simulink model "SIL_OlfatiSaber"  (R2021b)
settings: Solver=FixedStepDiscrete  StartTime=0  StopTime=T  FixedStep=0.01  RelTol=1e-3  EnableMultiTasking=on
model workspace (MAT data in the model file):
  SL_ROS_VariableLengthArrays_MaxSizes.CommonInfo.ArrayTruncateAction = 'EmitWarning'
  SL_ROS_VariableLengthArrays_MaxSizes.MsgTypeMap = containers.Map
  SL_ROS_VariableLengthArrays_MaxSizes.MsgTypeMap.serialization.keys = {'aircraft_communication/NetworkComm', 'aircraft_messages/Communication', 'aircraft_messages/NetworkComm', 'cosmus_messages/Communication', 'cosmus_messages/NetworkComm', 'cosmus_messages/WifiSignal', 'cosmus_messages/WifiSignals', 'sensor_msgs/Image'}
  SL_ROS_VariableLengthArrays_MaxSizes.MsgTypeMap.serialization.values{1}.PropertyName = 'Comms'
  SL_ROS_VariableLengthArrays_MaxSizes.MsgTypeMap.serialization.values{1}.DataType = 'aircraft_communication/Communication'
  SL_ROS_VariableLengthArrays_MaxSizes.MsgTypeMap.serialization.values{1}.MaxLength = 4
  SL_ROS_VariableLengthArrays_MaxSizes.MsgTypeMap.serialization.values{2}.PropertyName = 'Ssid'
  SL_ROS_VariableLengthArrays_MaxSizes.MsgTypeMap.serialization.values{2}.DataType = 'uint8'
  SL_ROS_VariableLengthArrays_MaxSizes.MsgTypeMap.serialization.values{2}.MaxLength = 6
  SL_ROS_VariableLengthArrays_MaxSizes.MsgTypeMap.serialization.values{3}.PropertyName = 'Comms'
  SL_ROS_VariableLengthArrays_MaxSizes.MsgTypeMap.serialization.values{3}.DataType = 'aircraft_messages/Communication'
  SL_ROS_VariableLengthArrays_MaxSizes.MsgTypeMap.serialization.values{3}.MaxLength = 4
  SL_ROS_VariableLengthArrays_MaxSizes.MsgTypeMap.serialization.values{4}.PropertyName = 'Ssid'
  SL_ROS_VariableLengthArrays_MaxSizes.MsgTypeMap.serialization.values{4}.DataType = 'uint8'
  SL_ROS_VariableLengthArrays_MaxSizes.MsgTypeMap.serialization.values{4}.MaxLength = 16
  SL_ROS_VariableLengthArrays_MaxSizes.MsgTypeMap.serialization.values{5}.PropertyName = 'Comms'
  SL_ROS_VariableLengthArrays_MaxSizes.MsgTypeMap.serialization.values{5}.DataType = 'cosmus_messages/Communication'
  SL_ROS_VariableLengthArrays_MaxSizes.MsgTypeMap.serialization.values{5}.MaxLength = 5
  SL_ROS_VariableLengthArrays_MaxSizes.MsgTypeMap.serialization.values{6}.PropertyName = 'Ssid'
  SL_ROS_VariableLengthArrays_MaxSizes.MsgTypeMap.serialization.values{6}.DataType = 'uint8'
  SL_ROS_VariableLengthArrays_MaxSizes.MsgTypeMap.serialization.values{6}.MaxLength = 1
  SL_ROS_VariableLengthArrays_MaxSizes.MsgTypeMap.serialization.values{7}.PropertyName = 'Signals'
  SL_ROS_VariableLengthArrays_MaxSizes.MsgTypeMap.serialization.values{7}.DataType = 'cosmus_messages/WifiSignal'
  SL_ROS_VariableLengthArrays_MaxSizes.MsgTypeMap.serialization.values{7}.MaxLength = 5
  SL_ROS_VariableLengthArrays_MaxSizes.MsgTypeMap.serialization.values{8}(1).PropertyName = 'Data'
  SL_ROS_VariableLengthArrays_MaxSizes.MsgTypeMap.serialization.values{8}(1).DataType = 'uint8'
  SL_ROS_VariableLengthArrays_MaxSizes.MsgTypeMap.serialization.values{8}(1).MaxLength = 259200
  SL_ROS_VariableLengthArrays_MaxSizes.MsgTypeMap.serialization.values{8}(2).PropertyName = 'Encoding'
  SL_ROS_VariableLengthArrays_MaxSizes.MsgTypeMap.serialization.values{8}(2).DataType = 'uint8'
  SL_ROS_VariableLengthArrays_MaxSizes.MsgTypeMap.serialization.values{8}(2).MaxLength = 259200
  SL_ROS_VariableLengthArrays_MaxSizes.MsgTypeMap.serialization.uniformity = 0
  SL_ROS_VariableLengthArrays_MaxSizes.MsgTypeMap.serialization.keyType = 'char'
  SL_ROS_VariableLengthArrays_MaxSizes.MsgTypeMap.serialization.valueType = 'any'
values from neighbouring files (symbols this model uses):
  airspeed_ref = 42    [start_swarm.m]
  altitude_ref = 300    [start_swarm.m]
  N_Waypoints = size(Waypoints,1)    [start_swarm.m]
  radius_waypoint = 200    [start_swarm.m]
  Waypoints = [1200 -1000 ... (first row only)    [start_swarm.m]
undefined symbols (not defined in the file or in its folder): DiscIntNeverNeededParam, Elevators, p_swarm, Propeller, RightAileron, RightFlap, Rudder
libraries: robotlib x36, slpidlib x15, eeGeneralControl x5, simulink x5
(part 1 of 5)
settings Model: Creator=fcsou  LastModifiedBy=fabricio
settings SolverCC: AlgebraicLoopSolver=TrustRegion
settings OptimizationCC: EnhancedBackFolding=on  PassReuseOutputArgsThreshold=0  MaxStackSize=64  OptimizeBlockOrder=speed  DifferentSizesBufferReuse=on  OptimizationCustomize=off
settings DebuggingCC: ParameterTunabilityLossMsg=error  SFMachineParentedDataDiag=warning
settings HardwareCC: ProdBitPerPointer=32  ProdBitPerSizeT=32  ProdBitPerPtrDiffT=32  ProdLargestAtomicFloat=None  ProdIntDivRoundTo=Undefined  ProdEndianess=Unspecified  ProdWordSize=32  ProdHWDeviceType=Generic->Unspecified (assume 32-bit Generic)  UseEmbeddedCoderFeatures=off
settings SFSimCC: MATLABDynamicMemAlloc=off
settings RTWCC: Description=Embedded Coder  SystemTargetFile=ert.tlc  HardwareBoard=Robot Operating System (ROS)  TLCOptions="-aInlineSetEventsForThisBaseRateFcn=TLC_FALSE -aSuppressMultiTaskScheduler=TLC_FALSE  -aRateBasedStepFcn=0"  TemplateMakefile=ert_default_tmf  Toolchain=Catkin  TargetLang=C++
settings CodeAppCC: ForceParamTrailComments=on  OperatorAnnotations=on
settings ERTTargetCC: ERTCustomFileBanners=off  SupportContinuousTime=on  SupportNonInlinedSFcns=on  RemoveResetFunc=off  ModelStepFunctionPrototypeControlCompliant=off  ERTCustomFileTemplate=rostime_codertarget_file_process.tlc

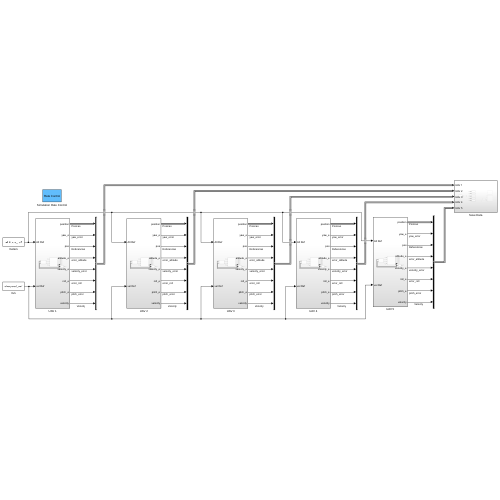
[thumbnail: Simulink's stored preview of the top-level diagram]
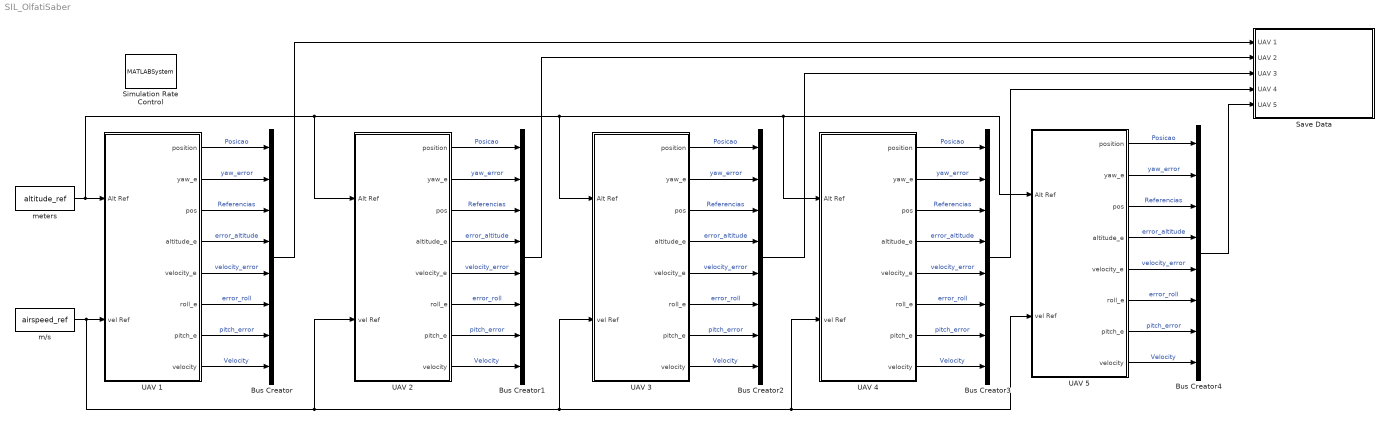
== system SIL_OlfatiSaber ==
  Bus Creator{,1..4} (5 alike) : BusCreator  Inputs=8
  Save Data : Subsystem
  Simulation Rate Control : MATLABSystem  System=ExampleHelperSimulationRateControl  SampleTime=0.01
      mask Type: ExampleHelperSimulationRateControl
      mask Display: disp('Rate Control');
  UAV 1 : Subsystem
  UAV 2 : Subsystem
  UAV 3 : Subsystem
  UAV 4 : Subsystem
  UAV 5 : Subsystem
  m/s : Constant  Value=airspeed_ref
  meters : Constant  Value=altitude_ref
  wires:
  UAV 1/1(position) -> Bus Creator/1  "Posicao"
  UAV 1/2(yaw_e) -> Bus Creator/2  "yaw_error"
  UAV 1/3(pos) -> Bus Creator/3  "Referencias"
  UAV 1/4(altitude_e) -> Bus Creator/4  "error_altitude"
  UAV 1/5(velocity_e) -> Bus Creator/5  "velocity_error"
  UAV 1/6(roll_e) -> Bus Creator/6  "error_roll"
  UAV 1/7(pitch_e) -> Bus Creator/7  "pitch_error"
  m/s/1 -> UAV 5/2(vel Ref), UAV 4/2(vel Ref), UAV 3/2(vel Ref), UAV 2/2(vel Ref), UAV 1/2(vel Ref)
  meters/1 -> UAV 5/1(Alt Ref), UAV 4/1(Alt Ref), UAV 3/1(Alt Ref), UAV 2/1(Alt Ref), UAV 1/1(Alt Ref)
  UAV 1/8(velocity) -> Bus Creator/8  "Velocity"
  UAV 2/7(pitch_e) -> Bus Creator1/7  "pitch_error"
  UAV 2/1(position) -> Bus Creator1/1  "Posicao"
  UAV 2/5(velocity_e) -> Bus Creator1/5  "velocity_error"
  UAV 2/3(pos) -> Bus Creator1/3  "Referencias"
  UAV 2/6(roll_e) -> Bus Creator1/6  "error_roll"
  UAV 2/8(velocity) -> Bus Creator1/8  "Velocity"
  UAV 2/4(altitude_e) -> Bus Creator1/4  "error_altitude"
  UAV 2/2(yaw_e) -> Bus Creator1/2  "yaw_error"
  UAV 3/5(velocity_e) -> Bus Creator2/5  "velocity_error"
  UAV 3/3(pos) -> Bus Creator2/3  "Referencias"
  UAV 3/7(pitch_e) -> Bus Creator2/7  "pitch_error"
  UAV 3/2(yaw_e) -> Bus Creator2/2  "yaw_error"
  UAV 3/6(roll_e) -> Bus Creator2/6  "error_roll"
  UAV 3/4(altitude_e) -> Bus Creator2/4  "error_altitude"
  UAV 3/8(velocity) -> Bus Creator2/8  "Velocity"
  UAV 3/1(position) -> Bus Creator2/1  "Posicao"
  Bus Creator/1 -> Save Data/1(UAV 1)
  Bus Creator1/1 -> Save Data/2(UAV 2)
  Bus Creator2/1 -> Save Data/3(UAV 3)
  UAV 4/4(altitude_e) -> Bus Creator3/4  "error_altitude"
  UAV 4/5(velocity_e) -> Bus Creator3/5  "velocity_error"
  UAV 4/7(pitch_e) -> Bus Creator3/7  "pitch_error"
  UAV 4/8(velocity) -> Bus Creator3/8  "Velocity"
  UAV 4/2(yaw_e) -> Bus Creator3/2  "yaw_error"
  UAV 4/3(pos) -> Bus Creator3/3  "Referencias"
  UAV 4/6(roll_e) -> Bus Creator3/6  "error_roll"
  UAV 4/1(position) -> Bus Creator3/1  "Posicao"
  UAV 5/4(altitude_e) -> Bus Creator4/4  "error_altitude"
  UAV 5/5(velocity_e) -> Bus Creator4/5  "velocity_error"
  UAV 5/7(pitch_e) -> Bus Creator4/7  "pitch_error"
  UAV 5/8(velocity) -> Bus Creator4/8  "Velocity"
  UAV 5/2(yaw_e) -> Bus Creator4/2  "yaw_error"
  UAV 5/3(pos) -> Bus Creator4/3  "Referencias"
  UAV 5/6(roll_e) -> Bus Creator4/6  "error_roll"
  UAV 5/1(position) -> Bus Creator4/1  "Posicao"
  Bus Creator3/1 -> Save Data/4(UAV 4)
  Bus Creator4/1 -> Save Data/5(UAV 5)

== system SIL_OlfatiSaber/Save Data ==
  UAV 1 : Inport
  UAV 2 : Inport  Port=2
  UAV 3 : Inport  Port=3
  UAV 4 : Inport  Port=4
  UAV 5 : Inport  Port=5
  Constant : Constant  Commented=on  Value=p_swarm.r
  Constant1 : Constant  Commented=on  Value=p_swarm.nb_agents
  Current Time : robotlib/Current Time  OutputFormat=double  SampleTime=-1  ModelName=SIL_OlfatiSaber
      settings: SourceProductBaseCode=RR
  Formation Shape Plot : MATLAB Function  Commented=on  TreatAsAtomicUnit=on
  Positions Plot : MATLAB Function  Commented=on  TreatAsAtomicUnit=on
  To Workspace1 : ToWorkspace  VariableName=UAV1  SaveFormat=Timeseries  SampleTime=-1
  To Workspace2 : ToWorkspace  VariableName=UAV2  SaveFormat=Timeseries  SampleTime=-1
  To Workspace3 : ToWorkspace  VariableName=UAV3  SaveFormat=Timeseries  SampleTime=-1
  To Workspace4 : ToWorkspace  VariableName=UAV4  SaveFormat=Timeseries  SampleTime=-1
  To Workspace5 : ToWorkspace  VariableName=UAV5  SaveFormat=Timeseries  SampleTime=-1
  To Workspace6 : ToWorkspace  VariableName=ROStime  SaveFormat=Timeseries  SampleTime=-1
  wires:
  UAV 1/1 -> To Workspace1/1
  UAV 3/1 -> To Workspace3/1
  UAV 4/1 -> To Workspace4/1
  UAV 5/1 -> To Workspace5/1
  Current Time/1 -> To Workspace6/1
  UAV 2/1 -> To Workspace2/1
  Constant/1 -> Formation Shape Plot/3(r_comm)
  Constant1/1 -> Formation Shape Plot/4(max_agent)

== system SIL_OlfatiSaber/UAV 1 ==
  Alt Ref : Inport
  vel Ref : Inport  Port=2
  Filtered Derivative (Discrete or Continuous) : eeGeneralControl/Filtered Derivative (Discrete or Continuous)  K=1  T=0.1  B=inf  A=-inf  minRatio=10  init_option=Inherited from block input  x0=0  Ts=-1
      settings: SourceProductBaseCode=PS
  High-level : Subsystem
  Low-level : Subsystem
  position : Outport
  yaw_e : Outport  Port=2
  pos : Outport  Port=3
  altitude_e : Outport  Port=4
  velocity_e : Outport  Port=5
  roll_e : Outport  Port=6
  pitch_e : Outport  Port=7
  velocity : Outport  Port=8
  wires:
  Low-level/7(position) -> High-level/1(Pos_I), Filtered Derivative (Discrete or Continuous)/1, position/1
  vel Ref/1 -> Low-level/1(vel ref)
  Alt Ref/1 -> Low-level/4(altitude ref)
  Low-level/1(alt_e) -> altitude_e/1
  Low-level/2(yaw_error) -> yaw_e/1
  Low-level/3(positions) -> pos/1
  Low-level/4(vel_e) -> velocity_e/1
  Low-level/5(roll_e) -> roll_e/1
  Low-level/6(pitch_e) -> pitch_e/1
  High-level/1(x ref) -> Low-level/2(x ref)
  High-level/2(y ref) -> Low-level/3(y ref)
  Low-level/8(Network) -> High-level/2(Network_Scan)
  Filtered Derivative (Discrete or Continuous)/1 -> velocity/1

== system SIL_OlfatiSaber/UAV 2 ==
  Alt Ref : Inport
  vel Ref : Inport  Port=2
  Filtered Derivative (Discrete or Continuous) : eeGeneralControl/Filtered Derivative (Discrete or Continuous)  K=1  T=0.1  B=inf  A=-inf  minRatio=10  init_option=Inherited from block input  x0=0  Ts=-1
      settings: SourceProductBaseCode=PS
  High-level : Subsystem
  Low-level : Subsystem
  position : Outport
  yaw_e : Outport  Port=2
  pos : Outport  Port=3
  altitude_e : Outport  Port=4
  velocity_e : Outport  Port=5
  roll_e : Outport  Port=6
  pitch_e : Outport  Port=7
  velocity : Outport  Port=8
  wires:
  Low-level/7(position) -> High-level/1(Pos_I), Filtered Derivative (Discrete or Continuous)/1, position/1
  vel Ref/1 -> Low-level/1(vel ref)
  Alt Ref/1 -> Low-level/4(altitude ref)
  Low-level/1(alt_e) -> altitude_e/1
  Low-level/2(yaw_error) -> yaw_e/1
  Low-level/3(positions) -> pos/1
  Low-level/4(vel_e) -> velocity_e/1
  Low-level/5(roll_e) -> roll_e/1
  Low-level/6(pitch_e) -> pitch_e/1
  High-level/1(x ref) -> Low-level/2(x ref)
  High-level/2(y ref) -> Low-level/3(y ref)
  Low-level/8(Network) -> High-level/2(Network_Scan)
  Filtered Derivative (Discrete or Continuous)/1 -> velocity/1

== system SIL_OlfatiSaber/UAV 3 ==
  Alt Ref : Inport
  vel Ref : Inport  Port=2
  Filtered Derivative (Discrete or Continuous) : eeGeneralControl/Filtered Derivative (Discrete or Continuous)  K=1  T=0.1  B=inf  A=-inf  minRatio=10  init_option=Inherited from block input  x0=0  Ts=-1
      settings: SourceProductBaseCode=PS
  High-level : Subsystem
  Low-level : Subsystem
  position : Outport
  yaw_e : Outport  Port=2
  pos : Outport  Port=3
  altitude_e : Outport  Port=4
  velocity_e : Outport  Port=5
  roll_e : Outport  Port=6
  pitch_e : Outport  Port=7
  velocity : Outport  Port=8
  wires:
  Low-level/7(position) -> Filtered Derivative (Discrete or Continuous)/1, High-level/1(Pos_I), position/1
  vel Ref/1 -> Low-level/1(vel ref)
  Alt Ref/1 -> Low-level/4(altitude ref)
  Low-level/1(alt_e) -> altitude_e/1
  Low-level/2(yaw_error) -> yaw_e/1
  Low-level/3(positions) -> pos/1
  Low-level/4(vel_e) -> velocity_e/1
  Low-level/5(roll_e) -> roll_e/1
  Low-level/6(pitch_e) -> pitch_e/1
  High-level/1(x ref) -> Low-level/2(x ref)
  High-level/2(y ref) -> Low-level/3(y ref)
  Low-level/8(Network) -> High-level/2(Network_Scan)
  Filtered Derivative (Discrete or Continuous)/1 -> velocity/1

== system SIL_OlfatiSaber/UAV 4 ==
  Alt Ref : Inport
  vel Ref : Inport  Port=2
  Filtered Derivative (Discrete or Continuous) : eeGeneralControl/Filtered Derivative (Discrete or Continuous)  K=1  T=0.1  B=inf  A=-inf  minRatio=10  init_option=Inherited from block input  x0=0  Ts=-1
      settings: SourceProductBaseCode=PS
  High-level : Subsystem
  Low-level : Subsystem
  position : Outport
  yaw_e : Outport  Port=2
  pos : Outport  Port=3
  altitude_e : Outport  Port=4
  velocity_e : Outport  Port=5
  roll_e : Outport  Port=6
  pitch_e : Outport  Port=7
  velocity : Outport  Port=8
  wires:
  Low-level/7(position) -> Filtered Derivative (Discrete or Continuous)/1, High-level/1(Pos_I), position/1
  vel Ref/1 -> Low-level/1(vel ref)
  Alt Ref/1 -> Low-level/4(altitude ref)
  Low-level/1(alt_e) -> altitude_e/1
  Low-level/2(yaw_error) -> yaw_e/1
  Low-level/3(positions) -> pos/1
  Low-level/4(vel_e) -> velocity_e/1
  Low-level/5(roll_e) -> roll_e/1
  Low-level/6(pitch_e) -> pitch_e/1
  High-level/1(x ref) -> Low-level/2(x ref)
  High-level/2(y ref) -> Low-level/3(y ref)
  Low-level/8(Network) -> High-level/2(Network_Scan)
  Filtered Derivative (Discrete or Continuous)/1 -> velocity/1

== system SIL_OlfatiSaber/UAV 5 ==
  Alt Ref : Inport
  vel Ref : Inport  Port=2
  Filtered Derivative (Discrete or Continuous) : eeGeneralControl/Filtered Derivative (Discrete or Continuous)  K=1  T=0.1  B=inf  A=-inf  minRatio=10  init_option=Inherited from block input  x0=0  Ts=-1
      settings: SourceProductBaseCode=PS
  High-level : Subsystem
  Low-level : Subsystem
  position : Outport
  yaw_e : Outport  Port=2
  pos : Outport  Port=3
  altitude_e : Outport  Port=4
  velocity_e : Outport  Port=5
  roll_e : Outport  Port=6
  pitch_e : Outport  Port=7
  velocity : Outport  Port=8
  wires:
  Low-level/7(position) -> Filtered Derivative (Discrete or Continuous)/1, High-level/1(Pos_I), position/1
  vel Ref/1 -> Low-level/1(vel ref)
  Alt Ref/1 -> Low-level/4(altitude ref)
  Low-level/1(alt_e) -> altitude_e/1
  Low-level/2(yaw_error) -> yaw_e/1
  Low-level/3(positions) -> pos/1
  Low-level/4(vel_e) -> velocity_e/1
  Low-level/5(roll_e) -> roll_e/1
  Low-level/6(pitch_e) -> pitch_e/1
  High-level/1(x ref) -> Low-level/2(x ref)
  High-level/2(y ref) -> Low-level/3(y ref)
  Low-level/8(Network) -> High-level/2(Network_Scan)
  Filtered Derivative (Discrete or Continuous)/1 -> velocity/1

== system SIL_OlfatiSaber/UAV 1/High-level ==
  Pos_I : Inport
  Network_Scan : Inport  Port=2
  Coordination Algorithm : Subsystem
  Network : Subsystem
  Terminator5 : Terminator
  Waypoint Generator : Subsystem
  x ref : Outport
  y ref : Outport  Port=2
  wires:
  Network/1(Pos_J) -> Coordination Algorithm/1(Xi), Waypoint Generator/1(Xi)
  Network_Scan/1 -> Network/1(Scan)
  Pos_I/1 -> Waypoint Generator/2(Pos_i)
  Coordination Algorithm/1(X) -> x ref/1
  Coordination Algorithm/2(Y) -> y ref/1
  Waypoint Generator/1(u) -> Coordination Algorithm/2(u)
  Coordination Algorithm/3(Z) -> Terminator5/1

== system SIL_OlfatiSaber/UAV 1/Low-level ==
  vel ref : Inport
  x ref : Inport  Port=2
  y ref : Inport  Port=3
  altitude ref : Inport  Port=4
  Autopilot : Subsystem
      settings: PortSchema="{\"entries\":[{\"content\":{\"sides\":[{\"content\":{\"connectorIds\":[\"In1\",\"In2\",\"In3\",\"In4\",\"In5\",\"In6\"]},\"type\":\"ConnectorPlacement.EquallySpacedRectSide\",\"uuid\":\"f5987fb5-26bd-460f-ada3-c62a2cc917d9\"},{\"content\":{\"connectorIds\":[\"Out1\",\"Out2\",\"Out3\",\"Out4\"],\"side\":\"RIGHT\"},\"type\":\"ConnectorPlacement.EquallySpacedRectSide\",\"uuid\":\"78b4fbb6-b2d6-45e8-a79e-ccfb1aa742fa\"},{\"content\":{\"connectorIds\":[\"Out5\",\"Out6\",\"Out7\",\"Out8\"],\"side\":\"TOP\"},\"type\":\"ConnectorPlacement.EquallySpacedRectSide\",\"uuid\":\"043ac8db-db42-42ba-ba46-d4f45f772f93\"},{\"content\":{\"connectorIds\":[],\"side\":\"HIDDEN\"},\"type\":\"ConnectorPlacement.EquallySpacedRectSide\",\"uuid\":\"557a5d68-6739-4613-818d-4b3751c4f08a\"}]},\"type\":\"ConnectorPlacement.EquallySpacedConnector\",\"uuid\":\"675ce67f-dd1b-4b16-8fb4-2c0be5e81414\"}],\"packageUris\":[\"http://schema.mathworks.com/mf0/Connector/R2020b\"],\"version\":\"1.0\"}"
  Bus Selector1 : BusSelector  OutputSignals=PositionX,PositionY
  Guidance Algorithm : Subsystem
      settings: PortSchema="{\"entries\":[{\"content\":{\"sides\":[{\"content\":{\"connectorIds\":[\"In1\",\"In2\",\"In3\",\"In4\",\"In5\"]},\"type\":\"ConnectorPlacement.EquallySpacedRectSide\",\"uuid\":\"b0b83658-dc10-4011-a234-ab17b261f867\"},{\"content\":{\"connectorIds\":[\"Out1\"],\"side\":\"RIGHT\"},\"type\":\"ConnectorPlacement.EquallySpacedRectSide\",\"uuid\":\"f99dae16-3a0a-4b7a-a248-8f98f89ef8fb\"},{\"content\":{\"connectorIds\":[\"Out2\",\"Out3\"],\"side\":\"TOP\"},\"type\":\"ConnectorPlacement.EquallySpacedRectSide\",\"uuid\":\"275bc05e-c915-4930-a6d1-ba5a3a506250\"},{\"content\":{\"connectorIds\":[],\"side\":\"HIDDEN\"},\"type\":\"ConnectorPlacement.EquallySpacedRectSide\",\"uuid\":\"a071ce22-c6e1-49a1-b318-d26a8e8cfe9f\"}]},\"type\":\"ConnectorPlacement.EquallySpacedConnector\",\"uuid\":\"e0998603-dd40-4b43-8488-1ee2e7350a27\"}],\"packageUris\":[\"http://schema.mathworks.com/mf0/Connector/R2020b\"],\"version\":\"1.0\"}"
  ROS Settings : Subsystem
  Vision : Subsystem
  alt_e : Outport
  yaw_error : Outport  Port=2
  positions : Outport  Port=3
  vel_e : Outport  Port=4
  roll_e : Outport  Port=5
  pitch_e : Outport  Port=6
  position : Outport  Port=7
  Network : Outport  Port=8
  wires:
  ROS Settings/2(Yaw) -> Guidance Algorithm/1(yaw)
  ROS Settings/5(velocity) -> Autopilot/5(vel_in)
  Guidance Algorithm/1(roll_ref) -> Autopilot/3(roll_ref)
  ROS Settings/1(Euler angles) -> Autopilot/2(Euler angles)
  Autopilot/8(pitch_e) -> pitch_e/1
  Autopilot/3(aileron_cmd) -> ROS Settings/3(ailerons)
  Autopilot/7(roll_e) -> roll_e/1
  Autopilot/1(profundor_cmd) -> ROS Settings/1(elevator)
  Autopilot/2(rudder_cmd) -> ROS Settings/2(rudder)
  Autopilot/4(propeller_cmd) -> ROS Settings/4(propeller)
  ROS Settings/4(altitude) -> Autopilot/4(altitude)
  Autopilot/5(alt_e) -> alt_e/1
  y ref/1 -> Guidance Algorithm/5(y ref)
  Autopilot/6(vel_e) -> vel_e/1
  vel ref/1 -> Autopilot/1(vel ref)
  Guidance Algorithm/3(positions) -> positions/1
  altitude ref/1 -> Autopilot/6(altitude ref)
  Guidance Algorithm/2(yaw_error) -> yaw_error/1
  x ref/1 -> Guidance Algorithm/4(x ref)
  Bus Selector1/2 -> Guidance Algorithm/3(y)  "<PositionY>"
  ROS Settings/3(position) -> position/1, Bus Selector1/1
  Bus Selector1/1 -> Guidance Algorithm/2(x)  "<PositionX>"
  ROS Settings/7(Image) -> Vision/1(Image)
  ROS Settings/6(wf_ij) -> Network/1

== system SIL_OlfatiSaber/UAV 2/High-level ==
  Pos_I : Inport
  Network_Scan : Inport  Port=2
  Coordination Algorithm : Subsystem
  Network : Subsystem
  Terminator5 : Terminator
  Waypoint Generator : Subsystem
  x ref : Outport
  y ref : Outport  Port=2
  wires:
  Network/1(Pos_J) -> Coordination Algorithm/1(Xi), Waypoint Generator/1(Xi)
  Network_Scan/1 -> Network/1(Scan)
  Pos_I/1 -> Waypoint Generator/2(Pos_i)
  Coordination Algorithm/1(X) -> x ref/1
  Coordination Algorithm/2(Y) -> y ref/1
  Waypoint Generator/1(u) -> Coordination Algorithm/2(u)
  Coordination Algorithm/3(Z) -> Terminator5/1

== system SIL_OlfatiSaber/UAV 2/Low-level ==
  vel ref : Inport
  x ref : Inport  Port=2
  y ref : Inport  Port=3
  altitude ref : Inport  Port=4
  Autopilot : Subsystem
      settings: PortSchema="{\"entries\":[{\"content\":{\"sides\":[{\"content\":{\"connectorIds\":[\"In1\",\"In2\",\"In3\",\"In4\",\"In5\",\"In6\"]},\"type\":\"ConnectorPlacement.EquallySpacedRectSide\",\"uuid\":\"f5987fb5-26bd-460f-ada3-c62a2cc917d9\"},{\"content\":{\"connectorIds\":[\"Out1\",\"Out2\",\"Out3\",\"Out4\"],\"side\":\"RIGHT\"},\"type\":\"ConnectorPlacement.EquallySpacedRectSide\",\"uuid\":\"78b4fbb6-b2d6-45e8-a79e-ccfb1aa742fa\"},{\"content\":{\"connectorIds\":[\"Out5\",\"Out6\",\"Out7\",\"Out8\"],\"side\":\"TOP\"},\"type\":\"ConnectorPlacement.EquallySpacedRectSide\",\"uuid\":\"043ac8db-db42-42ba-ba46-d4f45f772f93\"},{\"content\":{\"connectorIds\":[],\"side\":\"HIDDEN\"},\"type\":\"ConnectorPlacement.EquallySpacedRectSide\",\"uuid\":\"557a5d68-6739-4613-818d-4b3751c4f08a\"}]},\"type\":\"ConnectorPlacement.EquallySpacedConnector\",\"uuid\":\"675ce67f-dd1b-4b16-8fb4-2c0be5e81414\"}],\"packageUris\":[\"http://schema.mathworks.com/mf0/Connector/R2020b\"],\"version\":\"1.0\"}"
  Bus Selector1 : BusSelector  OutputSignals=PositionX,PositionY
  Guidance Algorithm : Subsystem
      settings: PortSchema="{\"entries\":[{\"content\":{\"sides\":[{\"content\":{\"connectorIds\":[\"In1\",\"In2\",\"In3\",\"In4\",\"In5\"]},\"type\":\"ConnectorPlacement.EquallySpacedRectSide\",\"uuid\":\"b0b83658-dc10-4011-a234-ab17b261f867\"},{\"content\":{\"connectorIds\":[\"Out1\"],\"side\":\"RIGHT\"},\"type\":\"ConnectorPlacement.EquallySpacedRectSide\",\"uuid\":\"f99dae16-3a0a-4b7a-a248-8f98f89ef8fb\"},{\"content\":{\"connectorIds\":[\"Out2\",\"Out3\"],\"side\":\"TOP\"},\"type\":\"ConnectorPlacement.EquallySpacedRectSide\",\"uuid\":\"275bc05e-c915-4930-a6d1-ba5a3a506250\"},{\"content\":{\"connectorIds\":[],\"side\":\"HIDDEN\"},\"type\":\"ConnectorPlacement.EquallySpacedRectSide\",\"uuid\":\"a071ce22-c6e1-49a1-b318-d26a8e8cfe9f\"}]},\"type\":\"ConnectorPlacement.EquallySpacedConnector\",\"uuid\":\"e0998603-dd40-4b43-8488-1ee2e7350a27\"}],\"packageUris\":[\"http://schema.mathworks.com/mf0/Connector/R2020b\"],\"version\":\"1.0\"}"
  ROS Settings : Subsystem
  Vision : Subsystem
  alt_e : Outport
  yaw_error : Outport  Port=2
  positions : Outport  Port=3
  vel_e : Outport  Port=4
  roll_e : Outport  Port=5
  pitch_e : Outport  Port=6
  position : Outport  Port=7
  Network : Outport  Port=8
  wires:
  ROS Settings/2(Yaw) -> Guidance Algorithm/1(yaw)
  ROS Settings/5(velocity) -> Autopilot/5(vel_in)
  Guidance Algorithm/1(roll_ref) -> Autopilot/3(roll_ref)
  ROS Settings/1(Euler angles) -> Autopilot/2(Euler angles)
  Autopilot/8(pitch_e) -> pitch_e/1
  Autopilot/3(aileron_cmd) -> ROS Settings/3(ailerons)
  Autopilot/7(roll_e) -> roll_e/1
  Autopilot/1(profundor_cmd) -> ROS Settings/1(elevator)
  Autopilot/2(rudder_cmd) -> ROS Settings/2(rudder)
  Autopilot/4(propeller_cmd) -> ROS Settings/4(propeller)
  ROS Settings/4(altitude) -> Autopilot/4(altitude)
  Autopilot/5(alt_e) -> alt_e/1
  y ref/1 -> Guidance Algorithm/5(y ref)
  Autopilot/6(vel_e) -> vel_e/1
  vel ref/1 -> Autopilot/1(vel ref)
  Guidance Algorithm/3(positions) -> positions/1
  altitude ref/1 -> Autopilot/6(altitude ref)
  Guidance Algorithm/2(yaw_error) -> yaw_error/1
  x ref/1 -> Guidance Algorithm/4(x ref)
  Bus Selector1/2 -> Guidance Algorithm/3(y)  "<PositionY>"
  ROS Settings/3(position) -> position/1, Bus Selector1/1
  Bus Selector1/1 -> Guidance Algorithm/2(x)  "<PositionX>"
  ROS Settings/7(Image) -> Vision/1(Image)
  ROS Settings/6(wf_ij) -> Network/1

== system SIL_OlfatiSaber/UAV 3/High-level ==
  Pos_I : Inport
  Network_Scan : Inport  Port=2
  Coordination Algorithm : Subsystem
  Network : Subsystem
  Terminator5 : Terminator
  Waypoint Generator : Subsystem
  x ref : Outport
  y ref : Outport  Port=2
  wires:
  Network/1(Pos_J) -> Coordination Algorithm/1(Xi), Waypoint Generator/1(Xi)
  Network_Scan/1 -> Network/1(Scan)
  Pos_I/1 -> Waypoint Generator/2(Pos_i)
  Coordination Algorithm/1(X) -> x ref/1
  Coordination Algorithm/2(Y) -> y ref/1
  Waypoint Generator/1(u) -> Coordination Algorithm/2(u)
  Coordination Algorithm/3(Z) -> Terminator5/1

== system SIL_OlfatiSaber/UAV 3/Low-level ==
  vel ref : Inport
  x ref : Inport  Port=2
  y ref : Inport  Port=3
  altitude ref : Inport  Port=4
  Autopilot : Subsystem
      settings: PortSchema="{\"entries\":[{\"content\":{\"sides\":[{\"content\":{\"connectorIds\":[\"In1\",\"In2\",\"In3\",\"In4\",\"In5\",\"In6\"]},\"type\":\"ConnectorPlacement.EquallySpacedRectSide\",\"uuid\":\"f5987fb5-26bd-460f-ada3-c62a2cc917d9\"},{\"content\":{\"connectorIds\":[\"Out1\",\"Out2\",\"Out3\",\"Out4\"],\"side\":\"RIGHT\"},\"type\":\"ConnectorPlacement.EquallySpacedRectSide\",\"uuid\":\"78b4fbb6-b2d6-45e8-a79e-ccfb1aa742fa\"},{\"content\":{\"connectorIds\":[\"Out5\",\"Out6\",\"Out7\",\"Out8\"],\"side\":\"TOP\"},\"type\":\"ConnectorPlacement.EquallySpacedRectSide\",\"uuid\":\"043ac8db-db42-42ba-ba46-d4f45f772f93\"},{\"content\":{\"connectorIds\":[],\"side\":\"HIDDEN\"},\"type\":\"ConnectorPlacement.EquallySpacedRectSide\",\"uuid\":\"557a5d68-6739-4613-818d-4b3751c4f08a\"}]},\"type\":\"ConnectorPlacement.EquallySpacedConnector\",\"uuid\":\"675ce67f-dd1b-4b16-8fb4-2c0be5e81414\"}],\"packageUris\":[\"http://schema.mathworks.com/mf0/Connector/R2020b\"],\"version\":\"1.0\"}"
  Bus Selector1 : BusSelector  OutputSignals=PositionX,PositionY
  Guidance Algorithm : Subsystem
      settings: PortSchema="{\"entries\":[{\"content\":{\"sides\":[{\"content\":{\"connectorIds\":[\"In1\",\"In2\",\"In3\",\"In4\",\"In5\"]},\"type\":\"ConnectorPlacement.EquallySpacedRectSide\",\"uuid\":\"b0b83658-dc10-4011-a234-ab17b261f867\"},{\"content\":{\"connectorIds\":[\"Out1\"],\"side\":\"RIGHT\"},\"type\":\"ConnectorPlacement.EquallySpacedRectSide\",\"uuid\":\"f99dae16-3a0a-4b7a-a248-8f98f89ef8fb\"},{\"content\":{\"connectorIds\":[\"Out2\",\"Out3\"],\"side\":\"TOP\"},\"type\":\"ConnectorPlacement.EquallySpacedRectSide\",\"uuid\":\"275bc05e-c915-4930-a6d1-ba5a3a506250\"},{\"content\":{\"connectorIds\":[],\"side\":\"HIDDEN\"},\"type\":\"ConnectorPlacement.EquallySpacedRectSide\",\"uuid\":\"a071ce22-c6e1-49a1-b318-d26a8e8cfe9f\"}]},\"type\":\"ConnectorPlacement.EquallySpacedConnector\",\"uuid\":\"e0998603-dd40-4b43-8488-1ee2e7350a27\"}],\"packageUris\":[\"http://schema.mathworks.com/mf0/Connector/R2020b\"],\"version\":\"1.0\"}"
  ROS Settings : Subsystem
  Vision : Subsystem
  alt_e : Outport
  yaw_error : Outport  Port=2
  positions : Outport  Port=3
  vel_e : Outport  Port=4
  roll_e : Outport  Port=5
  pitch_e : Outport  Port=6
  position : Outport  Port=7
  Network : Outport  Port=8
  wires:
  ROS Settings/2(Yaw) -> Guidance Algorithm/1(yaw)
  ROS Settings/5(velocity) -> Autopilot/5(vel_in)
  Guidance Algorithm/1(roll_ref) -> Autopilot/3(roll_ref)
  ROS Settings/1(Euler angles) -> Autopilot/2(Euler angles)
  Autopilot/8(pitch_e) -> pitch_e/1
  Autopilot/3(aileron_cmd) -> ROS Settings/3(ailerons)
  Autopilot/7(roll_e) -> roll_e/1
  Autopilot/1(profundor_cmd) -> ROS Settings/1(elevator)
  Autopilot/2(rudder_cmd) -> ROS Settings/2(rudder)
  Autopilot/4(propeller_cmd) -> ROS Settings/4(propeller)
  ROS Settings/4(altitude) -> Autopilot/4(altitude)
  Autopilot/5(alt_e) -> alt_e/1
  y ref/1 -> Guidance Algorithm/5(y ref)
  Autopilot/6(vel_e) -> vel_e/1
  vel ref/1 -> Autopilot/1(vel ref)
  Guidance Algorithm/3(positions) -> positions/1
  altitude ref/1 -> Autopilot/6(altitude ref)
  Guidance Algorithm/2(yaw_error) -> yaw_error/1
  x ref/1 -> Guidance Algorithm/4(x ref)
  Bus Selector1/2 -> Guidance Algorithm/3(y)  "<PositionY>"
  ROS Settings/3(position) -> position/1, Bus Selector1/1
  Bus Selector1/1 -> Guidance Algorithm/2(x)  "<PositionX>"
  ROS Settings/7(Image) -> Vision/1(Image)
  ROS Settings/6(wf_ij) -> Network/1

== system SIL_OlfatiSaber/UAV 4/High-level ==
  Pos_I : Inport
  Network_Scan : Inport  Port=2
  Coordination Algorithm : Subsystem
  Network : Subsystem
  Terminator5 : Terminator
  Waypoint Generator : Subsystem
  x ref : Outport
  y ref : Outport  Port=2
  wires:
  Network/1(Pos_J) -> Coordination Algorithm/1(Xi), Waypoint Generator/1(Xi)
  Network_Scan/1 -> Network/1(Scan)
  Pos_I/1 -> Waypoint Generator/2(Pos_i)
  Coordination Algorithm/1(X) -> x ref/1
  Coordination Algorithm/2(Y) -> y ref/1
  Waypoint Generator/1(u) -> Coordination Algorithm/2(u)
  Coordination Algorithm/3(Z) -> Terminator5/1

== system SIL_OlfatiSaber/UAV 4/Low-level ==
  vel ref : Inport
  x ref : Inport  Port=2
  y ref : Inport  Port=3
  altitude ref : Inport  Port=4
  Autopilot : Subsystem
      settings: PortSchema="{\"entries\":[{\"content\":{\"sides\":[{\"content\":{\"connectorIds\":[\"In1\",\"In2\",\"In3\",\"In4\",\"In5\",\"In6\"]},\"type\":\"ConnectorPlacement.EquallySpacedRectSide\",\"uuid\":\"f5987fb5-26bd-460f-ada3-c62a2cc917d9\"},{\"content\":{\"connectorIds\":[\"Out1\",\"Out2\",\"Out3\",\"Out4\"],\"side\":\"RIGHT\"},\"type\":\"ConnectorPlacement.EquallySpacedRectSide\",\"uuid\":\"78b4fbb6-b2d6-45e8-a79e-ccfb1aa742fa\"},{\"content\":{\"connectorIds\":[\"Out5\",\"Out6\",\"Out7\",\"Out8\"],\"side\":\"TOP\"},\"type\":\"ConnectorPlacement.EquallySpacedRectSide\",\"uuid\":\"043ac8db-db42-42ba-ba46-d4f45f772f93\"},{\"content\":{\"connectorIds\":[],\"side\":\"HIDDEN\"},\"type\":\"ConnectorPlacement.EquallySpacedRectSide\",\"uuid\":\"557a5d68-6739-4613-818d-4b3751c4f08a\"}]},\"type\":\"ConnectorPlacement.EquallySpacedConnector\",\"uuid\":\"675ce67f-dd1b-4b16-8fb4-2c0be5e81414\"}],\"packageUris\":[\"http://schema.mathworks.com/mf0/Connector/R2020b\"],\"version\":\"1.0\"}"
  Bus Selector1 : BusSelector  OutputSignals=PositionX,PositionY
  Guidance Algorithm : Subsystem
      settings: PortSchema="{\"entries\":[{\"content\":{\"sides\":[{\"content\":{\"connectorIds\":[\"In1\",\"In2\",\"In3\",\"In4\",\"In5\"]},\"type\":\"ConnectorPlacement.EquallySpacedRectSide\",\"uuid\":\"b0b83658-dc10-4011-a234-ab17b261f867\"},{\"content\":{\"connectorIds\":[\"Out1\"],\"side\":\"RIGHT\"},\"type\":\"ConnectorPlacement.EquallySpacedRectSide\",\"uuid\":\"f99dae16-3a0a-4b7a-a248-8f98f89ef8fb\"},{\"content\":{\"connectorIds\":[\"Out2\",\"Out3\"],\"side\":\"TOP\"},\"type\":\"ConnectorPlacement.EquallySpacedRectSide\",\"uuid\":\"275bc05e-c915-4930-a6d1-ba5a3a506250\"},{\"content\":{\"connectorIds\":[],\"side\":\"HIDDEN\"},\"type\":\"ConnectorPlacement.EquallySpacedRectSide\",\"uuid\":\"a071ce22-c6e1-49a1-b318-d26a8e8cfe9f\"}]},\"type\":\"ConnectorPlacement.EquallySpacedConnector\",\"uuid\":\"e0998603-dd40-4b43-8488-1ee2e7350a27\"}],\"packageUris\":[\"http://schema.mathworks.com/mf0/Connector/R2020b\"],\"version\":\"1.0\"}"
  ROS Settings : Subsystem
  Vision : Subsystem
  alt_e : Outport
  yaw_error : Outport  Port=2
  positions : Outport  Port=3
  vel_e : Outport  Port=4
  roll_e : Outport  Port=5
  pitch_e : Outport  Port=6
  position : Outport  Port=7
  Network : Outport  Port=8
  wires:
  ROS Settings/2(Yaw) -> Guidance Algorithm/1(yaw)
  ROS Settings/5(velocity) -> Autopilot/5(vel_in)
  Guidance Algorithm/1(roll_ref) -> Autopilot/3(roll_ref)
  ROS Settings/1(Euler angles) -> Autopilot/2(Euler angles)
  Autopilot/8(pitch_e) -> pitch_e/1
  Autopilot/3(aileron_cmd) -> ROS Settings/3(ailerons)
  Autopilot/7(roll_e) -> roll_e/1
  Autopilot/1(profundor_cmd) -> ROS Settings/1(elevator)
  Autopilot/2(rudder_cmd) -> ROS Settings/2(rudder)
  Autopilot/4(propeller_cmd) -> ROS Settings/4(propeller)
  ROS Settings/4(altitude) -> Autopilot/4(altitude)
  Autopilot/5(alt_e) -> alt_e/1
  y ref/1 -> Guidance Algorithm/5(y ref)
  Autopilot/6(vel_e) -> vel_e/1
  vel ref/1 -> Autopilot/1(vel ref)
  Guidance Algorithm/3(positions) -> positions/1
  altitude ref/1 -> Autopilot/6(altitude ref)
  Guidance Algorithm/2(yaw_error) -> yaw_error/1
  x ref/1 -> Guidance Algorithm/4(x ref)
  Bus Selector1/2 -> Guidance Algorithm/3(y)  "<PositionY>"
  ROS Settings/3(position) -> position/1, Bus Selector1/1
  Bus Selector1/1 -> Guidance Algorithm/2(x)  "<PositionX>"
  ROS Settings/7(Image) -> Vision/1(Image)
  ROS Settings/6(wf_ij) -> Network/1

== system SIL_OlfatiSaber/UAV 5/High-level ==
  Pos_I : Inport
  Network_Scan : Inport  Port=2
  Coordination Algorithm : Subsystem
  Network : Subsystem
  Terminator5 : Terminator
  Waypoint Generator : Subsystem
  x ref : Outport
  y ref : Outport  Port=2
  wires:
  Network/1(Pos_J) -> Coordination Algorithm/1(Xi), Waypoint Generator/1(Xi)
  Network_Scan/1 -> Network/1(Scan)
  Pos_I/1 -> Waypoint Generator/2(Pos_i)
  Coordination Algorithm/1(X) -> x ref/1
  Coordination Algorithm/2(Y) -> y ref/1
  Waypoint Generator/1(u) -> Coordination Algorithm/2(u)
  Coordination Algorithm/3(Z) -> Terminator5/1

== system SIL_OlfatiSaber/UAV 5/Low-level ==
  vel ref : Inport
  x ref : Inport  Port=2
  y ref : Inport  Port=3
  altitude ref : Inport  Port=4
  Autopilot : Subsystem
      settings: PortSchema="{\"entries\":[{\"content\":{\"sides\":[{\"content\":{\"connectorIds\":[\"In1\",\"In2\",\"In3\",\"In4\",\"In5\",\"In6\"]},\"type\":\"ConnectorPlacement.EquallySpacedRectSide\",\"uuid\":\"f5987fb5-26bd-460f-ada3-c62a2cc917d9\"},{\"content\":{\"connectorIds\":[\"Out1\",\"Out2\",\"Out3\",\"Out4\"],\"side\":\"RIGHT\"},\"type\":\"ConnectorPlacement.EquallySpacedRectSide\",\"uuid\":\"78b4fbb6-b2d6-45e8-a79e-ccfb1aa742fa\"},{\"content\":{\"connectorIds\":[\"Out5\",\"Out6\",\"Out7\",\"Out8\"],\"side\":\"TOP\"},\"type\":\"ConnectorPlacement.EquallySpacedRectSide\",\"uuid\":\"043ac8db-db42-42ba-ba46-d4f45f772f93\"},{\"content\":{\"connectorIds\":[],\"side\":\"HIDDEN\"},\"type\":\"ConnectorPlacement.EquallySpacedRectSide\",\"uuid\":\"557a5d68-6739-4613-818d-4b3751c4f08a\"}]},\"type\":\"ConnectorPlacement.EquallySpacedConnector\",\"uuid\":\"675ce67f-dd1b-4b16-8fb4-2c0be5e81414\"}],\"packageUris\":[\"http://schema.mathworks.com/mf0/Connector/R2020b\"],\"version\":\"1.0\"}"
  Bus Selector1 : BusSelector  OutputSignals=PositionX,PositionY
  Guidance Algorithm : Subsystem
      settings: PortSchema="{\"entries\":[{\"content\":{\"sides\":[{\"content\":{\"connectorIds\":[\"In1\",\"In2\",\"In3\",\"In4\",\"In5\"]},\"type\":\"ConnectorPlacement.EquallySpacedRectSide\",\"uuid\":\"b0b83658-dc10-4011-a234-ab17b261f867\"},{\"content\":{\"connectorIds\":[\"Out1\"],\"side\":\"RIGHT\"},\"type\":\"ConnectorPlacement.EquallySpacedRectSide\",\"uuid\":\"f99dae16-3a0a-4b7a-a248-8f98f89ef8fb\"},{\"content\":{\"connectorIds\":[\"Out2\",\"Out3\"],\"side\":\"TOP\"},\"type\":\"ConnectorPlacement.EquallySpacedRectSide\",\"uuid\":\"275bc05e-c915-4930-a6d1-ba5a3a506250\"},{\"content\":{\"connectorIds\":[],\"side\":\"HIDDEN\"},\"type\":\"ConnectorPlacement.EquallySpacedRectSide\",\"uuid\":\"a071ce22-c6e1-49a1-b318-d26a8e8cfe9f\"}]},\"type\":\"ConnectorPlacement.EquallySpacedConnector\",\"uuid\":\"e0998603-dd40-4b43-8488-1ee2e7350a27\"}],\"packageUris\":[\"http://schema.mathworks.com/mf0/Connector/R2020b\"],\"version\":\"1.0\"}"
  ROS Settings : Subsystem
  Vision : Subsystem
  alt_e : Outport
  yaw_error : Outport  Port=2
  positions : Outport  Port=3
  vel_e : Outport  Port=4
  roll_e : Outport  Port=5
  pitch_e : Outport  Port=6
  position : Outport  Port=7
  Network : Outport  Port=8
  wires:
  ROS Settings/2(Yaw) -> Guidance Algorithm/1(yaw)
  ROS Settings/5(velocity) -> Autopilot/5(vel_in)
  Guidance Algorithm/1(roll_ref) -> Autopilot/3(roll_ref)
  ROS Settings/1(Euler angles) -> Autopilot/2(Euler angles)
  Autopilot/8(pitch_e) -> pitch_e/1
  Autopilot/3(aileron_cmd) -> ROS Settings/3(ailerons)
  Autopilot/7(roll_e) -> roll_e/1
  Autopilot/1(profundor_cmd) -> ROS Settings/1(elevator)
  Autopilot/2(rudder_cmd) -> ROS Settings/2(rudder)
  Autopilot/4(propeller_cmd) -> ROS Settings/4(propeller)
  ROS Settings/4(altitude) -> Autopilot/4(altitude)
  Autopilot/5(alt_e) -> alt_e/1
  y ref/1 -> Guidance Algorithm/5(y ref)
  Autopilot/6(vel_e) -> vel_e/1
  vel ref/1 -> Autopilot/1(vel ref)
  Guidance Algorithm/3(positions) -> positions/1
  altitude ref/1 -> Autopilot/6(altitude ref)
  Guidance Algorithm/2(yaw_error) -> yaw_error/1
  x ref/1 -> Guidance Algorithm/4(x ref)
  Bus Selector1/2 -> Guidance Algorithm/3(y)  "<PositionY>"
  ROS Settings/3(position) -> position/1, Bus Selector1/1
  Bus Selector1/1 -> Guidance Algorithm/2(x)  "<PositionX>"
  ROS Settings/7(Image) -> Vision/1(Image)
  ROS Settings/6(wf_ij) -> Network/1

== system SIL_OlfatiSaber/UAV 1/High-level/Coordination Algorithm ==
  Xi : Inport
  u : Inport  Port=2
  Demux : Demux  Outputs=3
  Discrete Derivative : simulink/Discrete/Discrete Derivative  gainval=1.0  ICPrevScaledInput=0.0  OutMin=[]  OutMax=[]  OutDataType=fixdt(1, 16)  OutScaling=2^-10  DoSatur=off
  Discrete-Time Integrator : DiscreteIntegrator  SampleTime=-1  ICPrevOutput=DiscIntNeverNeededParam  ICPrevScaledInput=DiscIntNeverNeededParam
  Olfati-Saber Algorithm : MATLAB Function  TreatAsAtomicUnit=on
  Parameters : Subsystem
  dt : Constant  Value=0.01
  r_agent : Constant  Value=p_swarm.r_agent
  X : Outport
  Y : Outport  Port=2
  Z : Outport  Port=3
  wires:
  Olfati-Saber Algorithm/1(vel_command) -> Discrete-Time Integrator/1
  dt/1 -> Olfati-Saber Algorithm/5(dt)
  r_agent/1 -> Olfati-Saber Algorithm/6(r_agent)
  Discrete-Time Integrator/1 -> Demux/1
  Demux/2 -> Y/1
  Demux/1 -> X/1
  Demux/3 -> Z/1
  Discrete Derivative/1 -> Olfati-Saber Algorithm/3(vel)
  Parameters/1(p_swarm) -> Olfati-Saber Algorithm/1(p_swarm_par)
  Xi/1 -> Discrete Derivative/1, Olfati-Saber Algorithm/2(pos)
  u/1 -> Olfati-Saber Algorithm/4(u_ref)

== system SIL_OlfatiSaber/UAV 1/High-level/Network ==
  Scan : Inport
  Agents Number : Constant  Value=p_swarm.nb_agents
  Bus Selector : BusSelector  OutputSignals=Neighbors Odometry,Wi-Fi Scan
  Status Network : MATLAB Function  Commented=on  TreatAsAtomicUnit=on
  Terminator5 : Terminator
  Pos_J : Outport
  wires:
  Status Network/1(SignalDbms) -> Terminator5/1
  Agents Number/1 -> Status Network/1(N_Agents)
  Scan/1 -> Bus Selector/1
  Bus Selector/1 -> Pos_J/1  "<Neighbors Odometry>"
  Bus Selector/2 -> Status Network/2(Wifi_Scan)  "<Wi-Fi Scan>"

== system SIL_OlfatiSaber/UAV 1/High-level/Waypoint Generator ==
  Xi : Inport
  Pos_i : Inport  Port=2
  Constant : Constant  Value=radius_waypoint
  Constant1 : Constant  Value=Waypoints
  Constant2 : Constant  Value=N_Waypoints
  Constant3 : Constant  Value=p_swarm.r
  Display : Display
  Memory : Memory
  Velocity Direction : MATLAB Function  TreatAsAtomicUnit=on
  Waypoint Algorithm : MATLAB Function  TreatAsAtomicUnit=on
  u : Outport
  wires:
  Memory/1 -> Waypoint Algorithm/6("Current_Waypoint ")
  Constant1/1 -> Waypoint Algorithm/4(Waypoints)
  Xi/1 -> Waypoint Algorithm/1(Xi)
  Constant3/1 -> Waypoint Algorithm/3(p_swarm_r)
  Constant2/1 -> Waypoint Algorithm/5(N_Waypoints)
  Waypoint Algorithm/2(Current_Waypoint) -> Memory/1, Display/1
  Constant/1 -> Waypoint Algorithm/2(R)
  Pos_i/1 -> Velocity Direction/1(pos)
  Velocity Direction/1(u_ref) -> u/1
  Waypoint Algorithm/1(wp) -> Velocity Direction/2(wp)

== system SIL_OlfatiSaber/UAV 1/Low-level/Autopilot ==
  note: bota po
  vel ref : Inport
  Euler angles : Inport  Port=2
  roll_ref : Inport  Port=3
  altitude : Inport  Port=4
  vel_in : Inport  Port=5
  altitude ref : Inport  Port=6
  Altitude Control : Subsystem
      settings: PortSchema="{\"entries\":[{\"content\":{\"sides\":[{\"content\":{\"connectorIds\":[\"In1\",\"In2\"]},\"type\":\"ConnectorPlacement.EquallySpacedRectSide\",\"uuid\":\"98c80c82-2588-492a-897d-d133440579b3\"},{\"content\":{\"connectorIds\":[\"Out1\"],\"side\":\"RIGHT\"},\"type\":\"ConnectorPlacement.EquallySpacedRectSide\",\"uuid\":\"157fcffb-564d-4941-a636-42e4165df758\"},{\"content\":{\"connectorIds\":[\"Out2\"],\"side\":\"TOP\"},\"type\":\"ConnectorPlacement.EquallySpacedRectSide\",\"uuid\":\"44b57248-226e-45fd-814c-d7eb072c2d1f\"},{\"content\":{\"connectorIds\":[],\"side\":\"HIDDEN\"},\"type\":\"ConnectorPlacement.EquallySpacedRectSide\",\"uuid\":\"dff6d6ab-ae11-4516-9107-00b7ae45fb5b\"}]},\"type\":\"ConnectorPlacement.EquallySpacedConnector\",\"uuid\":\"b6a62117-e3d4-4c2a-a3b5-b134a2ba950a\"}],\"packageUris\":[\"http://schema.mathworks.com/mf0/Connector/R2020b\"],\"version\":\"1.0\"}"
  Attitude Control : Subsystem
  Constant : Constant  Value=0
  Saturation2 : Saturate  UpperLimit=0.0523599  LowerLimit=-0.0523599
  Saturation3 : Saturate  UpperLimit=0.8  LowerLimit=0.6
  Saturation4 : Saturate  UpperLimit=0.0523599  LowerLimit=-0.0523599
  Takeoff : Subsystem  Commented=on
  Velocity Control : Subsystem
      settings: PortSchema="{\"entries\":[{\"content\":{\"sides\":[{\"content\":{\"connectorIds\":[\"In1\",\"In2\"]},\"type\":\"ConnectorPlacement.EquallySpacedRectSide\",\"uuid\":\"98c80c82-2588-492a-897d-d133440579b3\"},{\"content\":{\"connectorIds\":[\"Out1\"],\"side\":\"RIGHT\"},\"type\":\"ConnectorPlacement.EquallySpacedRectSide\",\"uuid\":\"157fcffb-564d-4941-a636-42e4165df758\"},{\"content\":{\"connectorIds\":[\"Out2\"],\"side\":\"TOP\"},\"type\":\"ConnectorPlacement.EquallySpacedRectSide\",\"uuid\":\"44b57248-226e-45fd-814c-d7eb072c2d1f\"},{\"content\":{\"connectorIds\":[],\"side\":\"HIDDEN\"},\"type\":\"ConnectorPlacement.EquallySpacedRectSide\",\"uuid\":\"dff6d6ab-ae11-4516-9107-00b7ae45fb5b\"}]},\"type\":\"ConnectorPlacement.EquallySpacedConnector\",\"uuid\":\"b6a62117-e3d4-4c2a-a3b5-b134a2ba950a\"}],\"packageUris\":[\"http://schema.mathworks.com/mf0/Connector/R2020b\"],\"version\":\"1.0\"}"
  profundor_cmd : Outport
  rudder_cmd : Outport  Port=2
  aileron_cmd : Outport  Port=3
  propeller_cmd : Outport  Port=4
  alt_e : Outport  Port=5
  vel_e : Outport  Port=6
  roll_e : Outport  Port=7
  pitch_e : Outport  Port=8
  wires:
  vel ref/1 -> Velocity Control/1(Velocity Ref)
  altitude ref/1 -> Altitude Control/1(Altitude Ref)
  vel_in/1 -> Velocity Control/2(Velocity)
  Altitude Control/2(altitude_error) -> alt_e/1
  Velocity Control/2(velocity_error) -> vel_e/1
  Altitude Control/1(Pitch_ref) -> Attitude Control/1(Pitch Ref)
  roll_ref/1 -> Attitude Control/2(Roll_ref)
  Euler angles/1 -> Attitude Control/3(Euler angles)
  Attitude Control/1(pitch_error) -> pitch_e/1, Saturation4/1
  Attitude Control/2(roll_error) -> Saturation2/1, roll_e/1
  Velocity Control/1(propeller_cmd) -> Saturation3/1
  Saturation3/1 -> propeller_cmd/1
  Saturation2/1 -> aileron_cmd/1
  Saturation4/1 -> profundor_cmd/1
  altitude/1 -> Altitude Control/2(Altitude)
  Constant/1 -> rudder_cmd/1

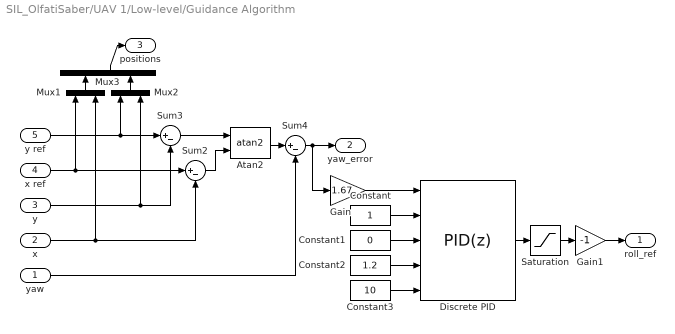
== system SIL_OlfatiSaber/UAV 1/Low-level/Guidance Algorithm ==
  yaw : Inport
  x : Inport  Port=2
  y : Inport  Port=3
  x ref : Inport  Port=4
  y ref : Inport  Port=5
  Atan2 : Trigonometry  Operator=atan2
  Constant : Constant
  Constant1 : Constant  Value=0
  Constant2 : Constant  Value=1.2
  Constant3 : Constant  Value=10
  Discrete PID : slpidlib/PID Controller  Controller=PID  Form=Parallel  TimeDomain=Discrete-time  UseExternalTs=off  SampleTime=-1  IntegratorMethod=Forward Euler  FilterMethod=Forward Euler  ControllerParametersSource=external  P=1  I=1  D=0  UseFilter=on  N=100  TunerSelectOption=Transfer Function Based (PID Tuner App)  InitialConditionSource=internal  InitialConditionForIntegrator=0  InitialConditionForFilter=0  DifferentiatorICPrevScaledInput=0  ExternalReset=none  TrackingMode=off  Kt=1  LimitOutput=off  SatLimitsSource=internal  UpperSaturationLimit=inf  LowerSaturationLimit=-inf  LinearizeAsGain=on  AntiWindupMode=none  Kb=1  POutMin=[]  POutMax=[]  IOutMin=[]  IOutMax=[]  DOutMin=[]  DOutMax=[]  NOutMin=[]  NOutMax=[]  SumOutMin=[]  SumOutMax=[]  SaturationOutMin=[]  SaturationOutMax=[]  PParamMin=[]  PParamMax=[]  IParamMin=[]  IParamMax=[]  DParamMin=[]  DParamMax=[]  NParamMin=[]  NParamMax=[]  KbParamMin=[]  KbParamMax=[]  KtParamMin=[]  KtParamMax=[]  KbOutMin=[]  KbOutMax=[]  KtOutMin=[]  KtOutMax=[]  IntegratorOutMin=[]  IntegratorOutMax=[]  FilterOutMin=[]  FilterOutMax=[]  SumI1OutMin=[]  SumI1OutMax=[]  SumI2OutMin=[]  SumI2OutMax=[]  SumI3OutMin=[]  SumI3OutMax=[]  SumI4OutMin=[]  SumI4OutMax=[]  SumDOutMin=[]  SumDOutMax=[]  DifferentiatorOutMin=[]  DifferentiatorOutMax=[]  FilterDiffOutCoefMin=[]  FilterDiffOutCoefMax=[]  ReciprocalOutMin=[]  ReciprocalOutMax=[]  SumDenOutMin=[]  SumDenOutMax=[]  SumNumOutMin=[]  SumNumOutMax=[]  DivideOutMin=[]  DivideOutMax=[]  UdiffTsProdOutMin=[]  UdiffTsProdOutMax=[]  NTsProdOutMin=[]  NTsProdOutMax=[]  UintegralTsProdOutMin=[]  UintegralTsProdOutMax=[]  UngainTsProdOutMin=[]  UngainTsProdOutMax=[]  IntegratorContinuousStateAttributes=''  IntegratorStateMustResolveToSignalObject=off  IntegratorRTWStateStorageClass=Auto  FilterContinuousStateAttributes=''  FilterStateMustResolveToSignalObject=off  FilterRTWStateStorageClass=Auto  ParallelPVariant=ExternalParameters  IdealPVariant=Disabled  IVariant=ExternalParameters  DVariant=ExternalParameters  IntegratorVariant=Discrete  SatVariant=Disabled  AWVariant=Passthrough  PCopyVariant=Disabled  TRVariant=Disabled  FdbkBlocksVariant=Forward  IdealPFdbkVariant=Disabled  SatFdbkVariant=Disabled  DerivativeFilterVariant=ForwardEulerFilter  NVariant=ExternalParameters  NCopyVariant=Disabled  FilterICVariant=InternalICsFilter  IntegratorICVariant=InternalICs  ExternalResetVariant=Disabled  TRSumVariant=Passthrough  SumFdbkVariant=Disabled  SumVariant=Sum_PID  TsampFilterVariant=InternalTs  TsampNgainVariant=Passthrough  TsampIntegralVariant=Passthrough  ExternalSaturationOutDataTypeStr=Inherit: Same as second input
  Gain : Gain  Gain=1.67
  Gain1 : Gain  Gain=-1
  Mux1 : Mux  Inputs=2
  Mux2 : Mux  Inputs=2
  Mux3 : Mux  Inputs=2
  Saturation : Saturate  UpperLimit=0.226893  LowerLimit=-0.226893
  Sum2 : Sum  Inputs=|+-
  Sum3 : Sum  Inputs=|+-
  Sum4 : Sum  Inputs=|+-
  roll_ref : Outport
  yaw_error : Outport  Port=2
  positions : Outport  Port=3
  wires:
  Mux1/1 -> Mux3/1
  Mux2/1 -> Mux3/2
  Saturation/1 -> Gain1/1
  Sum3/1 -> Atan2/1
  y/1 -> Sum3/2, Mux2/2
  y ref/1 -> Mux2/1, Sum3/1
  x ref/1 -> Mux1/1, Sum2/1
  x/1 -> Sum2/2, Mux1/2
  Sum2/1 -> Atan2/2
  Atan2/1 -> Sum4/1
  yaw/1 -> Sum4/2
  Mux3/1 -> positions/1
  Discrete PID/1 -> Saturation/1
  Sum4/1 -> yaw_error/1, Gain/1
  Gain1/1 -> roll_ref/1
  Constant/1 -> Discrete PID/2
  Constant1/1 -> Discrete PID/3
  Constant2/1 -> Discrete PID/4
  Constant3/1 -> Discrete PID/5
  Gain/1 -> Discrete PID/1

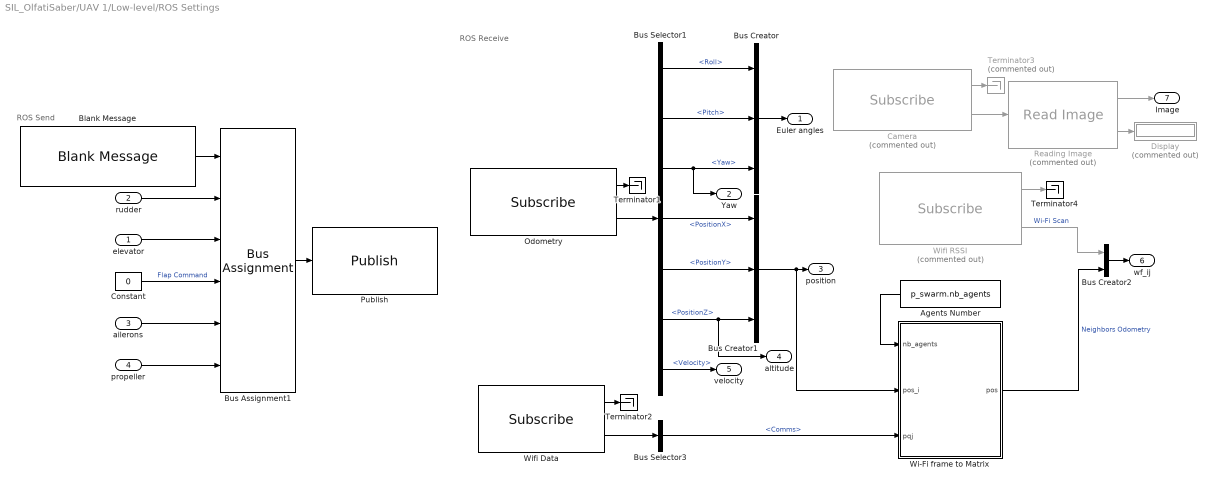
== system SIL_OlfatiSaber/UAV 1/Low-level/ROS Settings ==
  note: ROS Receive
  note: ROS Send
  elevator : Inport
  rudder : Inport  Port=2
  ailerons : Inport  Port=3
  propeller : Inport  Port=4
  Agents Number : Constant  Value=p_swarm.nb_agents
  Blank Message : robotlib/Blank Message  messageClass=Message  entityType=cosmus_messages/Control_Surfaces  messageType=cosmus_messages/Control_Surfaces  SampleTime=-1  legacyBusStruct=off
  Bus Assignment1 : BusAssignment  AssignedSignals=Rudder,Elevators,RightFlap,RightAileron,Propeller
  Bus Creator : BusCreator  Inputs=3
  Bus Creator1 : BusCreator  Inputs=3
  Bus Creator2 : BusCreator  Inputs=2
  Bus Selector1 : BusSelector  OutputSignals=Roll,Pitch,Yaw,PositionX,PositionY,PositionZ,Velocity
  Bus Selector3 : BusSelector  OutputSignals=Comms
  Camera : robotlib/Subscribe  Commented=on  topicSource=Select from ROS network  topic=/uav1/camera/image_raw  messageType=sensor_msgs/Image  SampleTime=-1  legacyBusStruct=off  messageQueueLength=1
  Constant : Constant  Value=0
  Display : Display  Commented=on
  Odometry : robotlib/Subscribe  topicSource=Select from ROS network  topic=/uav1/ground_truth/Odometry  messageType=cosmus_communication/Odom  SampleTime=-1  legacyBusStruct=off  messageQueueLength=1
  Publish : robotlib/Publish  topicSource=Select from ROS network  topic=/uav1/command  messageType=cosmus_messages/Control_Surfaces  legacyBusStruct=off  messageQueueLength=1
  Reading Image : robotlib/Read Image  Commented=on  MaximumImageSize=[240, 360]  ImageEncoding=rgb8  ShowAlphaOutput=off  ShowErrorCodeOutput=on  VariableSizeOutputs=off
      settings: SourceProductBaseCode=RR
  Terminator1 : Terminator
  Terminator2 : Terminator
  Terminator3 : Terminator  Commented=on
  Terminator4 : Terminator
  Wi-Fi frame to Matrix : MATLAB Function  TreatAsAtomicUnit=on
  Wifi Data : robotlib/Subscribe  topicSource=Select from ROS network  topic=/uav1/wifi_receiver/data  messageType=cosmus_messages/NetworkComm  SampleTime=-1  legacyBusStruct=off  messageQueueLength=1
  Wifi RSSI : robotlib/Subscribe  Commented=on  topicSource=Select from ROS network  topic=/uav1/wifi_receiver/wifi_scan  messageType=cosmus_messages/WifiSignals  SampleTime=-1  legacyBusStruct=off  messageQueueLength=1
  Euler angles : Outport
  Yaw : Outport  Port=2
  position : Outport  Port=3
  altitude : Outport  Port=4
  velocity : Outport  Port=5
  wf_ij : Outport  Port=6
  Image : Outport  Port=7
  wires:
  Odometry/1 -> Terminator1/1
  Blank Message/1 -> Bus Assignment1/1
  Bus Selector1/3 -> Bus Creator/3, Yaw/1  "<Yaw>"
  Bus Creator/1 -> Euler angles/1
  Bus Selector1/1 -> Bus Creator/1  "<Roll>"
  Bus Selector1/2 -> Bus Creator/2  "<Pitch>"
  Constant/1 -> Bus Assignment1/4  "Flap Command"
  Bus Assignment1/1 -> Publish/1
  Odometry/2 -> Bus Selector1/1
  Bus Selector1/4 -> Bus Creator1/1  "<PositionX>"
  Bus Selector1/5 -> Bus Creator1/2  "<PositionY>"
  Bus Selector1/6 -> Bus Creator1/3, altitude/1  "<PositionZ>"
  propeller/1 -> Bus Assignment1/6
  ailerons/1 -> Bus Assignment1/5
  elevator/1 -> Bus Assignment1/3
  Bus Selector1/7 -> velocity/1  "<Velocity>"
  rudder/1 -> Bus Assignment1/2
  Wifi Data/1 -> Terminator2/1
  Wifi Data/2 -> Bus Selector3/1
  Bus Selector3/1 -> Wi-Fi frame to Matrix/3(pqj)  "<Comms>"
  Agents Number/1 -> Wi-Fi frame to Matrix/1(nb_agents)
  Bus Creator1/1 -> position/1, Wi-Fi frame to Matrix/2(pos_i)
  Wi-Fi frame to Matrix/1(pos) -> Bus Creator2/2  "Neighbors Odometry"
  Camera/2 -> Reading Image/1
  Reading Image/1 -> Image/1
  Reading Image/2 -> Display/1
  Camera/1 -> Terminator3/1
  Wifi RSSI/1 -> Terminator4/1
  Wifi RSSI/2 -> Bus Creator2/1  "Wi-Fi Scan"
  Bus Creator2/1 -> wf_ij/1

== system SIL_OlfatiSaber/UAV 1/Low-level/Vision ==
  Image : Inport
  Video Viewer : VideoViewer  Commented=on  FigPos=[505 744 418 304]
  wires:
  Image/1 -> Video Viewer/1

== system SIL_OlfatiSaber/UAV 2/High-level/Coordination Algorithm ==
  Xi : Inport
  u : Inport  Port=2
  Demux : Demux  Outputs=3
  Discrete Derivative : simulink/Discrete/Discrete Derivative  gainval=1.0  ICPrevScaledInput=0.0  OutMin=[]  OutMax=[]  OutDataType=fixdt(1, 16)  OutScaling=2^-10  DoSatur=off
  Discrete-Time Integrator : DiscreteIntegrator  SampleTime=-1  ICPrevOutput=DiscIntNeverNeededParam  ICPrevScaledInput=DiscIntNeverNeededParam
  Olfati-Saber Algorithm : MATLAB Function  TreatAsAtomicUnit=on
  Parameters : Subsystem
  dt : Constant  Value=0.01
  r_agent : Constant  Value=p_swarm.r_agent
  X : Outport
  Y : Outport  Port=2
  Z : Outport  Port=3
  wires:
  Olfati-Saber Algorithm/1(vel_command) -> Discrete-Time Integrator/1
  dt/1 -> Olfati-Saber Algorithm/5(dt)
  r_agent/1 -> Olfati-Saber Algorithm/6(r_agent)
  Discrete-Time Integrator/1 -> Demux/1
  Demux/2 -> Y/1
  Demux/1 -> X/1
  Demux/3 -> Z/1
  Discrete Derivative/1 -> Olfati-Saber Algorithm/3(vel)
  Parameters/1(p_swarm) -> Olfati-Saber Algorithm/1(p_swarm_par)
  Xi/1 -> Discrete Derivative/1, Olfati-Saber Algorithm/2(pos)
  u/1 -> Olfati-Saber Algorithm/4(u_ref)

== system SIL_OlfatiSaber/UAV 2/High-level/Network ==
  Scan : Inport
  Agents Number : Constant  Value=p_swarm.nb_agents
  Bus Selector : BusSelector  OutputSignals=Neighbors Odometry,Wi-Fi Scan
  Status Network : MATLAB Function  Commented=on  TreatAsAtomicUnit=on
  Terminator5 : Terminator
  Pos_J : Outport
  wires:
  Status Network/1(SignalDbms) -> Terminator5/1
  Agents Number/1 -> Status Network/1(N_Agents)
  Scan/1 -> Bus Selector/1
  Bus Selector/1 -> Pos_J/1  "<Neighbors Odometry>"
  Bus Selector/2 -> Status Network/2(Wifi_Scan)  "<Wi-Fi Scan>"
